simulink model "UAV_Task_1"  (R2024b)
settings: Solver=ode45  StartTime=0.0  StopTime=100  FixedStep=1/1000  MaxStep=0.001  RelTol=1e-3
values from neighbouring files (symbols this model uses):
  k_f = 0.3379e-6    (= 3.379e-07)    [UAV_Task_1_main.m]
  Omega_0 = Omega_cmd    [UAV_Task_1_main.m]
  Omega_cmd = mean(trimedOmega)*ones(4,1)    [UAV_Task_1_main.m]
  omegab_0 = [0 0 0]'    [UAV_Task_1_main.m]
  p_0 = [0 0 -2]'    [UAV_Task_1_main.m]
  q_0 = rotm2quat(R_0)'    [UAV_Task_1_main.m]
  vb_0 = [0 0 0]'    [UAV_Task_1_main.m]
undefined symbols (not defined in the file or in its folder): Environment, UAV
settings Model: Creator=justs  LastModifiedBy=giuseppe
settings OptimizationCC: ReuseModelBlockBuffer=off
settings ModelReferenceCC: EnableRefExpFcnMdlSchedulingChecks=on
settings RTWCC: GPUComputeCapability=3.5

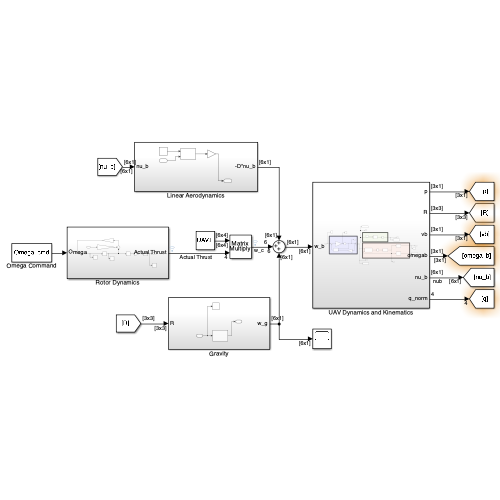
[thumbnail: Simulink's stored preview of the top-level diagram]
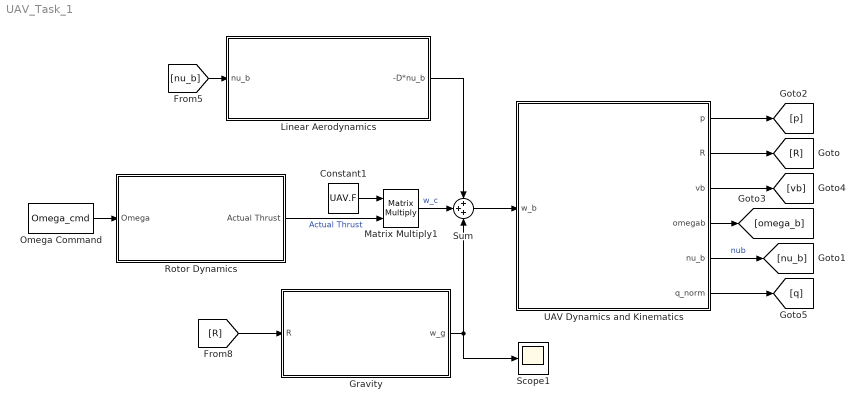
== system UAV_Task_1 ==
  Constant1 : Constant  Value=UAV.F
  Gravity : Subsystem
  Linear Aerodynamics : Subsystem
  Matrix Multiply1 : Product  Multiplication=Matrix(*)
  Omega Command : Constant  Value=Omega_cmd
  Rotor Dynamics : Subsystem
  Scope1 : Scope
  Sum : Sum  Inputs=+++
  UAV Dynamics and Kinematics : Subsystem
  wires:
  Sum/1 -> UAV Dynamics and Kinematics/1(w_b)
  Constant1/1 -> Matrix Multiply1/1
  Matrix Multiply1/1 -> Sum/2  "w_c"
  Rotor Dynamics/1(Actual Thrust) -> Matrix Multiply1/2  "Actual Thrust"
  UAV Dynamics and Kinematics/2(R) -> [R]
  UAV Dynamics and Kinematics/4(omegab) -> [omega_b]
  Linear Aerodynamics/1(-D*nu_b) -> Sum/1
  Gravity/1(w_g) -> Sum/3, Scope1/1
  UAV Dynamics and Kinematics/1(p) -> [p]
  UAV Dynamics and Kinematics/3(vb) -> [vb]
  UAV Dynamics and Kinematics/6(q_norm) -> [q]
  [nu_b] -> Linear Aerodynamics/1(nu_b)
  UAV Dynamics and Kinematics/5(nu_b) -> [nu_b]  "nub"
  [R] -> Gravity/1(R)
  Omega Command/1 -> Rotor Dynamics/1(Omega)

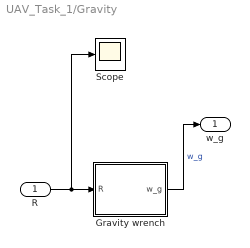
== system UAV_Task_1/Gravity ==
  R : Inport
  Gravity wrench : MATLAB Function  TreatAsAtomicUnit=on
  Scope : Scope
  w_g : Outport
  wires:
  Gravity wrench/1(w_g) -> w_g/1  "w_g"
  R/1 -> Scope/1, Gravity wrench/1(R)

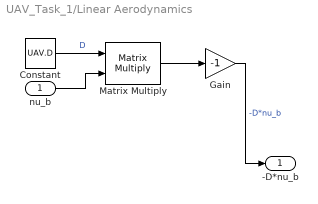
== system UAV_Task_1/Linear Aerodynamics ==
  nu_b : Inport
  Constant : Constant  Value=UAV.D
  Gain : Gain  Gain=-1
  Matrix Multiply : Product  Multiplication=Matrix(*)
  -D*nu_b : Outport
  wires:
  Gain/1 -> -D*nu_b/1  "-D*nu_b"
  Matrix Multiply/1 -> Gain/1
  Constant/1 -> Matrix Multiply/1  "D"
  nu_b/1 -> Matrix Multiply/2

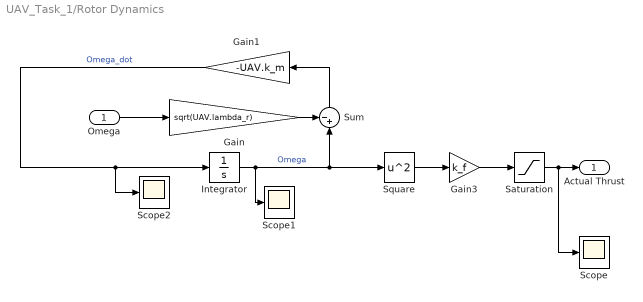
== system UAV_Task_1/Rotor Dynamics ==
  Omega : Inport
  Gain : Gain  Gain=sqrt(UAV.lambda_r)
  Gain1 : Gain  Gain=-UAV.k_m
  Gain3 : Gain  Gain=k_f
  Integrator : Integrator  InitialCondition=Omega_0
  Saturation : Saturate  UpperLimit=UAV.T_max  LowerLimit=UAV.T_min
  Scope : Scope
  Scope1 : Scope
  Scope2 : Scope
  Square : Math  Operator=square
  Sum : Sum  Inputs=-+|
  Actual Thrust : Outport
  wires:
  Square/1 -> Gain3/1
  Gain3/1 -> Saturation/1
  Saturation/1 -> Scope/1, Actual Thrust/1
  Omega/1 -> Gain/1
  Integrator/1 -> Scope1/1, Square/1, Sum/2  "Omega"
  Gain/1 -> Sum/1
  Sum/1 -> Gain1/1
  Gain1/1 -> Integrator/1, Scope2/1  "Omega_dot"

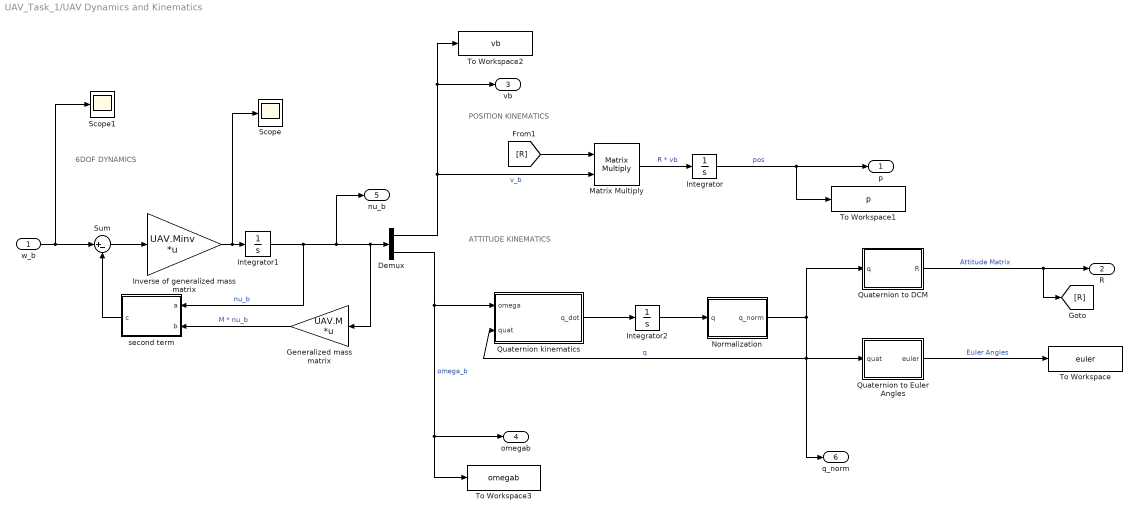
== system UAV_Task_1/UAV Dynamics and Kinematics ==
  note: 6DOF DYNAMICS
  note: ATTITUDE KINEMATICS
  note: POSITION KINEMATICS
  w_b : Inport
  Demux : Demux  Outputs=2
  Generalized mass matrix : Gain  Gain=UAV.M  Multiplication=Matrix(K*u)
  Integrator : Integrator  InitialCondition=p_0
  Integrator1 : Integrator  InitialCondition=[vb_0;omegab_0]
  Integrator2 : Integrator  InitialCondition=q_0
  Inverse of generalized mass matrix : Gain  Gain=UAV.Minv  Multiplication=Matrix(K*u)
  Matrix Multiply : Product  Multiplication=Matrix(*)
  Normalization : MATLAB Function  TreatAsAtomicUnit=on
  Quaternion kinematics : MATLAB Function  TreatAsAtomicUnit=on
  Quaternion to DCM : MATLAB Function  TreatAsAtomicUnit=on
  Quaternion to Euler Angles : MATLAB Function  TreatAsAtomicUnit=on
  Scope : Scope
  Scope1 : Scope
  Sum : Sum  Inputs=|+-
  To Workspace : ToWorkspace  VariableName=euler  SaveFormat=Timeseries  SampleTime=-1
  To Workspace1 : ToWorkspace  VariableName=p  SaveFormat=Timeseries  SampleTime=-1
  To Workspace2 : ToWorkspace  VariableName=vb  SaveFormat=Timeseries  SampleTime=-1
  To Workspace3 : ToWorkspace  VariableName=omegab  SaveFormat=Timeseries  SampleTime=-1
  "second term " : MATLAB Function  TreatAsAtomicUnit=on
  p : Outport
  R : Outport  Port=2
  vb : Outport  Port=3
  omegab : Outport  Port=4
  nu_b : Outport  Port=5
  q_norm : Outport  Port=6
  wires:
  Integrator/1 -> p/1, To Workspace1/1  "pos"
  Quaternion kinematics/1(q_dot) -> Integrator2/1
  Normalization/1(q_norm) -> q_norm/1, Quaternion kinematics/2(quat), Quaternion to Euler Angles/1(quat), Quaternion to DCM/1(q)  "q"
  Quaternion to DCM/1(R) -> R/1, [R]  "Attitude Matrix"
  Demux/1 -> Matrix Multiply/2, vb/1, To Workspace2/1  "v_b"
  Integrator1/1 -> nu_b/1, Demux/1, Generalized mass matrix/1, "second term "/1(a)  "nu_b"
  Integrator2/1 -> Normalization/1(q)
  Matrix Multiply/1 -> Integrator/1  "R * vb"
  Quaternion to Euler Angles/1(euler) -> To Workspace/1  "Euler Angles"
  [R] -> Matrix Multiply/1
  Inverse of generalized mass matrix/1 -> Scope/1, Integrator1/1
  Demux/2 -> omegab/1, To Workspace3/1, Quaternion kinematics/1(omega)  "omega_b"
  Generalized mass matrix/1 -> "second term "/2(b)  "M * nu_b"
  Sum/1 -> Inverse of generalized mass matrix/1
  "second term "/1(c) -> Sum/2
  w_b/1 -> Scope1/1, Sum/1

== matlab function UAV_Task_1/UAV Dynamics and Kinematics/Quaternion to Euler Angles ==
  data: quat input; euler output
function euler = quatToEuler( quat )
%	Converts a quaternion vector to ZYX Euler angles (RPY)

euler = quat2eul(quat','XYZ');

end

== matlab function UAV_Task_1/UAV Dynamics and Kinematics/Normalization ==
  data: q input; q_norm output
function q_norm = quat_norm( q )

norm = sqrt( q(1)^2 + q(2)^2 + q(3)^2 + q(4)^2 );

q_norm = 1/norm * q;

== matlab function UAV_Task_1/UAV Dynamics and Kinematics/Quaternion to DCM ==
  data: q input; R output
function R = fcn(q)

R = quat2rotm(q');

end

== matlab function UAV_Task_1/UAV Dynamics and Kinematics/second term  ==
  data: a input; c output; b input
function c = cross_six(a,b)

a_v = a(1:3);
a_omega = a(4:6);

cross_six = [crossmat(a_omega), zeros(3,3);
             crossmat(a_v), crossmat(a_omega)] ;

c = cross_six*b;

end

function S=crossmat(s)
S=[0  -s(3)  s(2);
    s(3)   0 -s(1);
    -s(2)  s(1)  0];
end

== matlab function UAV_Task_1/Gravity/Gravity wrench ==
  data: R input; w_g output; UAV parameter; Environment parameter
function w_g = fcn(R,UAV,Environment)

e_3 = Environment.e_3;
g = Environment.g;

w_g = g*[UAV.m*R'*e_3; UAV.S*R'*e_3];

== matlab function UAV_Task_1/UAV Dynamics and Kinematics/Quaternion kinematics ==
  data: omega input; quat input; q_dot output
 function q_dot = quat_kin(omega, quat)
%#codegen

eta = quat(1);
eps = quat(2:4);

W=[-eps';
   skew(eps) + eta*eye(3)];

q_dot = 0.5*W*omega;

end

function S=skew(s)
S=[0  -s(3)  s(2);
    s(3)   0 -s(1);
    -s(2)  s(1)  0];
end
